simulink model "sistema_real"  (R2015a)
settings: Solver=ode45  StartTime=0.0  StopTime=10.0  RelTol=1e-3
values from neighbouring files (symbols this model uses):
  A = [2.8883370741 1 0 0 0 -2.75968400411 0 1 0 0 0.525095601237 0 ... (25 elements, 5x5)]    [model_matrix_data424.mat]
  B = [1 0 0 0 0]    [model_matrix_data424.mat]
  C = [-0.0748175001742 0.149096420272 0 0 0]    [model_matrix_data424.mat]
  N = Ny+K*Nx    [lab4script.m]    (also in test_different_R.m; teste_sistema_real.m)
  Ts = 0.02    [lab4script.m]    (also in test_different_R.m; teste_sistema_real.m)
undefined symbols (not defined in the file or in its folder): K, Ke, Kp, M, MIO, National_Instruments, PCI
libraries: sldrtlib x2
settings Model: Creator=Margarida  LastModifiedBy=Margarida

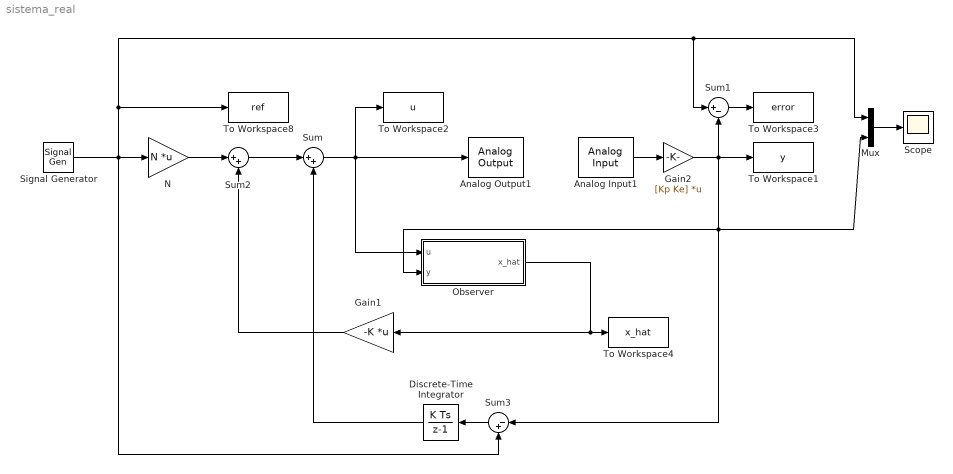
== system sistema_real ==
  Analog Input1 : sldrtlib/Analog Input  SampleTime=0.02  MaxMissedTicks=10  ShowMissedTicks=off  YieldWhenWaiting=off  DrvName=National_Instruments/PCI-MIO-16E-4  DrvAddress=4294967295  DrvOptions=[0 0 0 0 0 0]  Channels=[1 2]  RangeMode=1  VoltRange=1  DataType=1
      settings: AttributesFormatString=National Instruments\nPCI-MIO-16E-4 [auto]
  Analog Output1 : sldrtlib/Analog Output  SampleTime=0.02  MaxMissedTicks=10  ShowMissedTicks=off  YieldWhenWaiting=off  DrvName=National_Instruments/PCI-MIO-16E-4  DrvAddress=4294967295  DrvOptions=[0 0 0 0 0 0]  Channels=1  RangeMode=1  VoltRange=1  InitialValue=0  FinalValue=0
      settings: AttributesFormatString=National Instruments\nPCI-MIO-16E-4 [auto]
  Discrete-Time Integrator : DiscreteIntegrator  gainval=0.055  InitialConditionSetting=State (most efficient)  SampleTime=Ts
  Gain1 : Gain  Gain=-K  Multiplication=Matrix(K*u)
  Gain2 : Gain  Gain=[Kp Ke]  Multiplication=Matrix(K*u)
  Mux : Mux  Inputs=2
  N : Gain  Gain=N  Multiplication=Matrix(K*u)
  Observer : Subsystem
  Scope : Scope
      settings: YMin=-35  YMax=30
  Signal Generator : SignalGenerator  WaveForm=square  Amplitude=30  Frequency=0.1
  Sum : Sum  Inputs=|++
  Sum1 : Sum  Inputs=|+-
  Sum2 : Sum  Inputs=|++
  Sum3 : Sum  Inputs=|-+
  To Workspace1 : ToWorkspace  VariableName=y  SaveFormat=Structure With Time  SampleTime=Ts
  To Workspace2 : ToWorkspace  VariableName=u  SaveFormat=Structure With Time  SampleTime=Ts
  To Workspace3 : ToWorkspace  VariableName=error  SampleTime=Ts
  To Workspace4 : ToWorkspace  VariableName=x_hat  SaveFormat=Structure With Time  SampleTime=Ts
  To Workspace8 : ToWorkspace  VariableName=ref  SaveFormat=Structure With Time  SampleTime=Ts
  wires:
  Observer/1(x_hat) -> Gain1/1, To Workspace4/1
  Sum/1 -> Analog Output1/1, To Workspace2/1, Observer/1(u)
  Signal Generator/1 -> Sum3/2, N/1, Sum1/1, Mux/1, To Workspace8/1
  Sum1/1 -> To Workspace3/1
  Analog Input1/1 -> Gain2/1
  Gain2/1 -> Sum1/2, Sum3/1, Observer/2(y), Mux/2, To Workspace1/1
  Mux/1 -> Scope/1
  Sum2/1 -> Sum/1
  N/1 -> Sum2/1
  Discrete-Time Integrator/1 -> Sum/2
  Gain1/1 -> Sum2/2
  Sum3/1 -> Discrete-Time Integrator/1

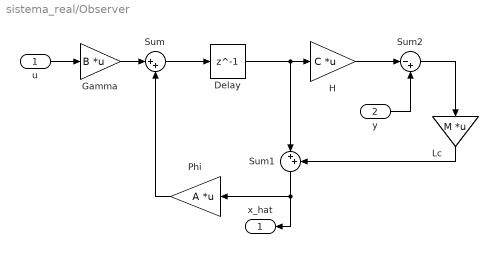
== system sistema_real/Observer ==
  u : Inport
  y : Inport  Port=2
  Delay : Delay  DelayLength=1  InitialCondition=0  SampleTime=Ts
  Gamma : Gain  Gain=B  Multiplication=Matrix(K*u)
  H : Gain  Gain=C  Multiplication=Matrix(K*u)
  Lc : Gain  Gain=M  Multiplication=Matrix(K*u)
  "Phi " : Gain  Gain=A  Multiplication=Matrix(K*u)
  Sum : Sum  Inputs=|++
  Sum1 : Sum  Inputs=|++
  Sum2 : Sum  Inputs=|-+
  x_hat : Outport
  wires:
  Gamma/1 -> Sum/1
  Sum/1 -> Delay/1
  Delay/1 -> Sum1/1, H/1
  "Phi "/1 -> Sum/2
  Sum1/1 -> x_hat/1, "Phi "/1
  H/1 -> Sum2/1
  Sum2/1 -> Lc/1
  Lc/1 -> Sum1/2
  u/1 -> Gamma/1
  y/1 -> Sum2/2
